simulink model "Lab6_2017B5A30983P_Fullwave_Controlled"  (R2019b)
settings: Solver=ode15s  StartTime=0.0  StopTime=0.1  RelTol=1e-3
libraries: powerlib x11, powerlib_meascontrol x2
settings Model: Creator=swaga  LastModifiedBy=swaga

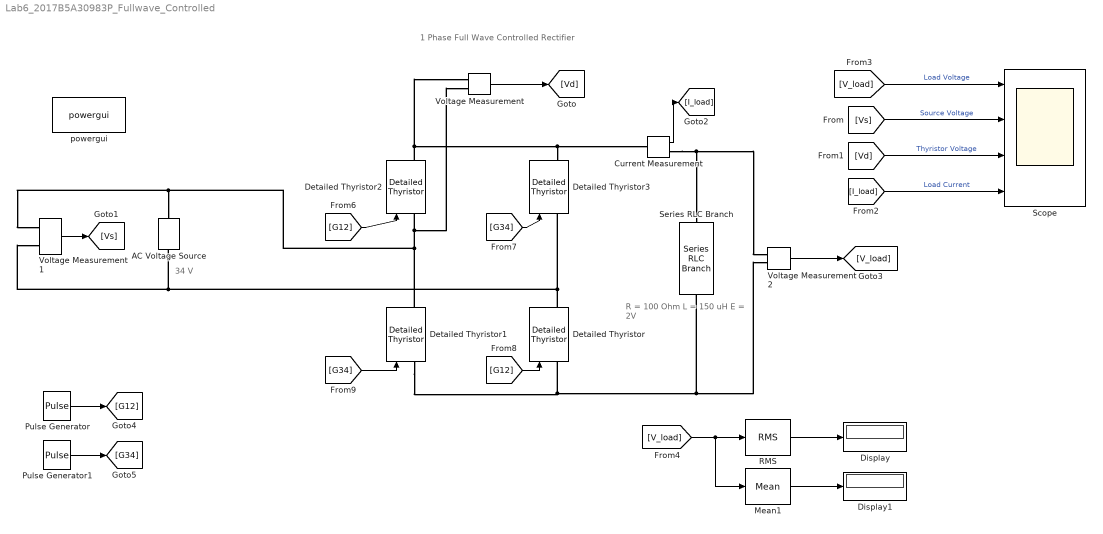
== system Lab6_2017B5A30983P_Fullwave_Controlled ==
  note: 1 Phase Full Wave Controlled Rectifier
  note: R = 100 Ohm
      | L =  150 uH
      | E = 2V
  note: 34 V
  AC Voltage Source : powerlib/Electrical Sources/AC Voltage Source  Amplitude=34  Phase=0  Frequency=50  SampleTime=0  Measurements=None  BusType=swing  Pref=10e3  Qref=0  Qmin=-inf  Qmax=+inf
      settings: SourceProductName=Simscape Electrical
  Current Measurement : powerlib/Measurements/Current Measurement  PhasorSimulation=off  OutputType=Complex  PSBequivalent=0
      settings: SourceProductName=Simscape Electrical
  Detailed Thyristor{,1..3} (4 alike) : powerlib/Power Electronics/Detailed Thyristor  Ron=0.001  Lon=1e-3  Vf=0.8  IL=0.1  Tq=100e-6  IC=0  Rs=500  Cs=250e-9  Measurements=on
      settings: SourceProductName=Simscape Electrical  SourceProductBaseCode=PS
  Display : Display
  Display1 : Display
  Mean1 : powerlib_meascontrol/Measurements/Mean  Freq=50  Vinit=0  Ts=0
      settings: SourceProductName=Simscape Electrical
  Pulse Generator : DiscretePulseGenerator  PulseType=Time based  Period=0.02  PulseWidth=5  PhaseDelay=0.0033
  Pulse Generator1 : DiscretePulseGenerator  PulseType=Time based  Period=0.02  PulseWidth=5  PhaseDelay=0.0133
  RMS : powerlib_meascontrol/Measurements/RMS  TrueRMS=on  Freq=50  RMSInit=120  Ts=0
      settings: SourceProductName=Simscape Electrical
  Scope : Scope  NumInputPorts=4
  Series RLC Branch : powerlib/Elements/Series RLC Branch  LConnTagsString=__new0  RConnTagsString=__new0  BranchType=R  Resistance=100  Inductance=1e-3  SetiL0=off  InitialCurrent=0  Capacitance=1e-6  Setx0=off  InitialVoltage=0  Measurements=None
      settings: SourceProductName=Simscape Electrical
  Voltage Measurement : powerlib/Measurements/Voltage Measurement  PhasorSimulation=off  OutputType=Complex  PSBequivalent=0
      settings: SourceProductName=Simscape Electrical
  Voltage Measurement1 : powerlib/Measurements/Voltage Measurement  PhasorSimulation=off  OutputType=Complex  PSBequivalent=0
      settings: SourceProductName=Simscape Electrical
  Voltage Measurement2 : powerlib/Measurements/Voltage Measurement  PhasorSimulation=off  OutputType=Complex  PSBequivalent=0
      settings: SourceProductName=Simscape Electrical
  powergui : powerlib/powergui  Priority=1  SimulationMode=Continuous  SampleTime=50e-6  frequency=60  Iterations=50  frequencyindice=50  Pbase=100e6  ErrMax=1e-4  UnitsV=kV  UnitsW=MW  buscounter=0  FunctionMessages=off  echomessages=off  EnableUseOfTLC=off  CurrentSourceSwitches=off  DisableSnubberDevices=off  DisableRonSwitches=off  DisableVfSwitches=off  DisplayEquations=off  AutomaticDiscreteSolvers=off  SolverType=Tustin/Backward Euler (TBE)  Interpol=off  ExternalGateDelay=off  methode=off  Ts=100  x0status=blocks  SPID=on  SwTol=0  HookPort=off  NonlinearTolerance=1e-4  nMaxIteration=100  ContinueOnMaxIteration=off  RestoreLinks=warning  ResistiveCurrentMeasurement=off  Frange=[0:2:500]  Ylog=off  Xlog=on  ShowGrid=off  save=off  variable=ZData  structure=0  ZoomFFT=off  StartTime=0.0  cycles=1  DisplayStyle=1  fundamental=60  FreqAxis=off  MaxFrequency=1000  frequencyindicesteady=1  RmsSteady=1  display=off
      settings: SourceProductName=Simscape Electrical
  wires:
  Voltage Measurement/1 -> [Vd]
  Voltage Measurement1/1 -> [Vs]
  Current Measurement/1 -> [I_load]
  Voltage Measurement2/1 -> [V_load]
  Pulse Generator1/1 -> [G34]
  Pulse Generator/1 -> [G12]
  [G12] -> Detailed Thyristor2/1
  [G12] -> Detailed Thyristor/1
  [G34] -> Detailed Thyristor3/1
  [G34] -> Detailed Thyristor1/1
  [V_load] -> Mean1/1, RMS/1
  RMS/1 -> Display/1
  Mean1/1 -> Display1/1
  [I_load] -> Scope/4  "Load Current"
  [Vd] -> Scope/3  "Thyristor Voltage"
  [Vs] -> Scope/2  "Source Voltage"
  [V_load] -> Scope/1  "Load Voltage"
  connections:
  Detailed Thyristor1/RConn1 -- AC Voltage Source/RConn1 -- Voltage Measurement1/LConn1 -- Voltage Measurement/LConn2 -- Detailed Thyristor2/LConn1
  Detailed Thyristor/RConn1 -- Detailed Thyristor3/LConn1 -- Voltage Measurement1/LConn2 -- AC Voltage Source/LConn1
  Detailed Thyristor1/LConn1 -- Voltage Measurement2/LConn2 -- Series RLC Branch/RConn1 -- Detailed Thyristor/LConn1
  Detailed Thyristor2/RConn1 -- Voltage Measurement/LConn1 -- Current Measurement/LConn1 -- Detailed Thyristor3/RConn1
  Current Measurement/RConn1 -- Series RLC Branch/LConn1 -- Voltage Measurement2/LConn1
